simulink model "CSTD1_ClosedLoopLQG"  (Simulink 8.9)
settings: Solver=ode5  StartTime=0.0  StopTime=15  FixedStep=0.001  RelTol=1e-3  EnableMultiTasking=on
values from neighbouring files (symbols this model uses):
  dist_on = 1    [CSTD1_LQGdesign.m]
  F = zeros(1,6)    [CSTD1_LQGdesign.m]
  F2 = Fi(1:6)    [CSTD1_LQGdesign.m]
  Ki = Fi(7)    [CSTD1_LQGdesign.m]
  L = -lqr(A',C3',Q_lqe,R_lqe)'    [CSTD1_LQGdesign.m]
  LQG_activation = 0    [CSTD1_LQGdesign.m]
  pre_v = 0    [CSTD1_LQGdesign.m]
undefined symbols (not defined in the file or in its folder): A, B, C, D
libraries: simulink x1
settings Model: Creator=jb  LastModifiedBy=AMG
settings DataIOCC: ExternalInput=[t, Plant_input_u]  LimitDataPoints=off  MaxDataPoints=20000  SaveOutput=off
settings OptimizationCC: BlockReduction=off  ExpressionDepthLimit=2147483647
settings DebuggingCC: SolverPrmCheckMsg=warning
settings ConfigComp: CovSFcnEnable=off

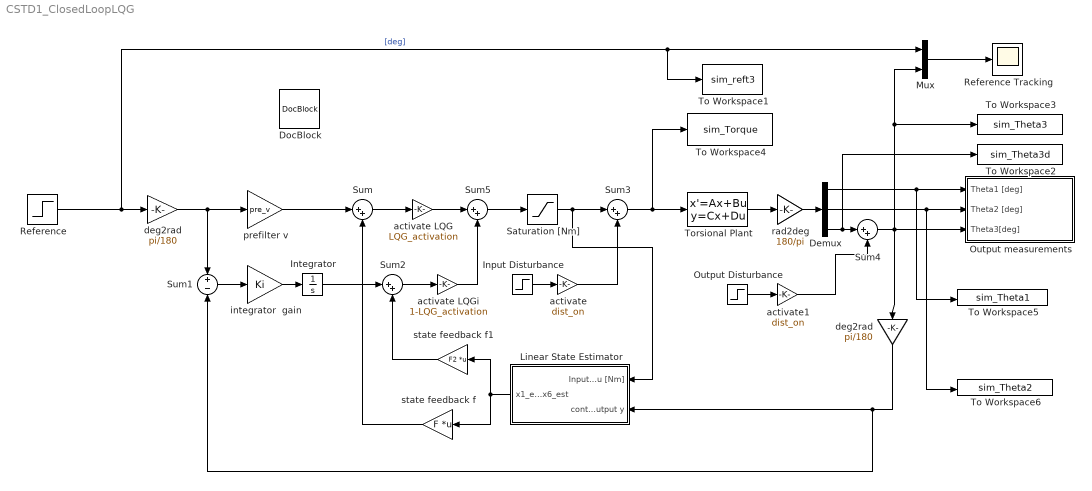
== system CSTD1_ClosedLoopLQG ==
  " deg2rad " : Gain  Gain=pi/180
  Demux : Demux  Outputs=3
  DocBlock : simulink/Model-Wide Utilities/DocBlock  DocumentType=Text
      content=|
      | % #########################################################################
      | % TUHH :: Institute for Control Systems :: Control Lab
      | % #########################################################################
      | % Experiment CSTD1: Control and Identification of a Torsional Plant
      | %
      | % Copyright Herbert Werner and Hamburg University of Technology, 2014
      | % #########################################################################
      | % This is the model containing the closed loop simulation for the LQG
      | % controllers design.
      | %
      | % Further, the following variables need to be in the workspace to run the
      | % experiment:
      | %  - pre_v   [double] : static prefilter
      | %  - F       [double] : standard state feedback gain
      | %  - L       [double] : observer gain
      | %  - F2      [double] : state feedback gain with integrator
      | %  - Ki      [double] : integrator gain
      | %  - A,B,C,D [double] : system matrices
      | %  - dist_on [double] : disturbance activation
      | %  - LQG_activation [double] : LQG switch
      | %
      | %----------------------------
      | % v.1.0 - 15-11-2014
      | % by Antonio Mendez G
  Input Disturbance : Step  Time=7  After=0.2  SampleTime=0
  Integrator : Integrator
  Linear State Estimator : Subsystem
  Mux : Mux  Inputs=2
  Output Disturbance : Step  Time=4  After=30  SampleTime=0
  Output measurements : Subsystem
  Reference : Step  Time=0  After=360  SampleTime=0
  Reference Tracking : Scope
  Saturation [Nm] : Saturate  UpperLimit=5*0.387  LowerLimit=-5*0.387
  Sum{,2..5} (5 alike) : Sum  Inputs=|++
  Sum1 : Sum  Inputs=+-
  To Workspace1 : ToWorkspace  VariableName=sim_reft3  SampleTime=-1
  To Workspace2 : ToWorkspace  VariableName=sim_Theta3d  SampleTime=-1
  To Workspace3 : ToWorkspace  VariableName=sim_Theta3  SampleTime=-1
  To Workspace4 : ToWorkspace  VariableName=sim_Torque  SampleTime=-1
  To Workspace5 : ToWorkspace  VariableName=sim_Theta1  SampleTime=-1
  To Workspace6 : ToWorkspace  VariableName=sim_Theta2  SampleTime=-1
  Torsional Plant : StateSpace  A=A  B=B  C=C  D=D  X0=[0 0.1 0 0.2 0 0.2]
  activate : Gain  Gain=dist_on
  activate LQG : Gain  Gain=LQG_activation
  activate LQGi : Gain  Gain=1-LQG_activation
  activate1 : Gain  Gain=dist_on
  deg2rad : Gain  Gain=pi/180
  integrator  gain : Gain  Gain=Ki
  prefilter v : Gain  Gain=pre_v
  rad2deg : Gain  Gain=180/pi
  state feedback f : Gain  Gain=F  Multiplication=Matrix(K*u) (u vector)
  state feedback f1 : Gain  Gain=F2  Multiplication=Matrix(K*u) (u vector)
  wires:
  Linear State Estimator/1(x1_est...x6_est) -> state feedback f1/1, state feedback f/1
  " deg2rad "/1 -> prefilter v/1, Sum1/1
  Reference/1 -> " deg2rad "/1, To Workspace1/1, Mux/1  "[deg]"
  rad2deg/1 -> Demux/1
  Torsional Plant/1 -> rad2deg/1
  state feedback f/1 -> Sum/2
  Mux/1 -> Reference Tracking/1
  Demux/2 -> To Workspace6/1, Output measurements/2(Theta2 [deg])
  Sum1/1 -> integrator  gain/1
  integrator  gain/1 -> Integrator/1
  deg2rad/1 -> Sum1/2, Linear State Estimator/2(control output y)
  Sum/1 -> activate LQG/1
  Integrator/1 -> Sum2/1
  state feedback f1/1 -> Sum2/2
  Sum2/1 -> activate LQGi/1
  Demux/1 -> To Workspace5/1, Output measurements/1(Theta1 [deg])
  Sum3/1 -> Torsional Plant/1, To Workspace4/1
  Saturation [Nm]/1 -> Linear State Estimator/1(Input u [Nm]), Sum3/1
  Output Disturbance/1 -> activate1/1
  Input Disturbance/1 -> activate/1
  activate/1 -> Sum3/2
  activate LQG/1 -> Sum5/1
  activate LQGi/1 -> Sum5/2
  Sum5/1 -> Saturation [Nm]/1
  prefilter v/1 -> Sum/1
  activate1/1 -> Sum4/2
  Demux/3 -> To Workspace2/1, Sum4/1
  Sum4/1 -> deg2rad/1, To Workspace3/1, Mux/2, Output measurements/3(Theta3[deg])

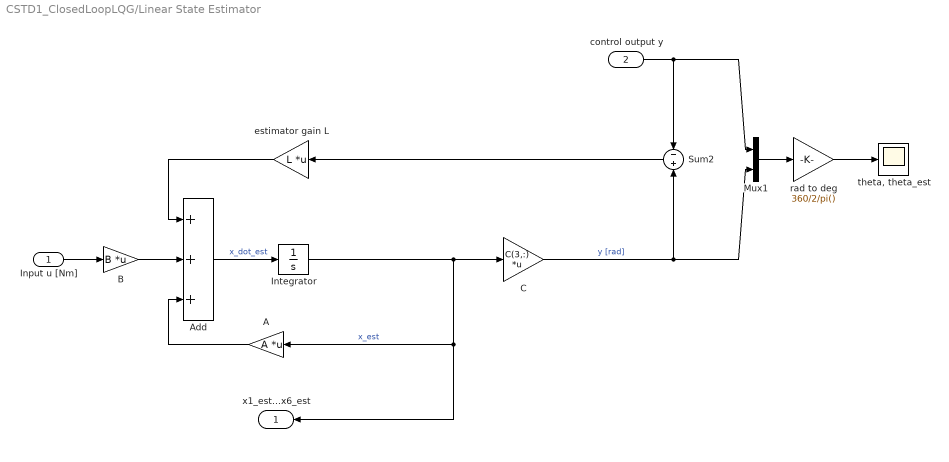
== system CSTD1_ClosedLoopLQG/Linear State Estimator ==
  Input u [Nm] : Inport
  control output y : Inport  Port=2
  " estimator gain L" : Gain  Gain=L  Multiplication=Matrix(K*u) (u vector)
  A : Gain  Gain=A  Multiplication=Matrix(K*u) (u vector)
  Add : Sum  Inputs=+++
  B : Gain  Gain=B  Multiplication=Matrix(K*u) (u vector)
  C : Gain  Gain=C(3,:)  Multiplication=Matrix(K*u) (u vector)
  Integrator : Integrator
  Mux1 : Mux  Inputs=2
  Sum2 : Sum  Inputs=-|+
  rad to deg : Gain  Gain=360/2/pi()
  "theta, theta_est" : Scope
  x1_est...x6_est : Outport
  wires:
  Input u [Nm]/1 -> B/1
  control output y/1 -> Sum2/1, Mux1/1
  Add/1 -> Integrator/1  "x_dot_est"
  Integrator/1 -> C/1, x1_est...x6_est/1, A/1  "x_est"
  C/1 -> Sum2/2, Mux1/2  "y [rad]"
  Mux1/1 -> rad to deg/1
  rad to deg/1 -> "theta, theta_est"/1
  " estimator gain L"/1 -> Add/1
  B/1 -> Add/2
  A/1 -> Add/3
  Sum2/1 -> " estimator gain L"/1

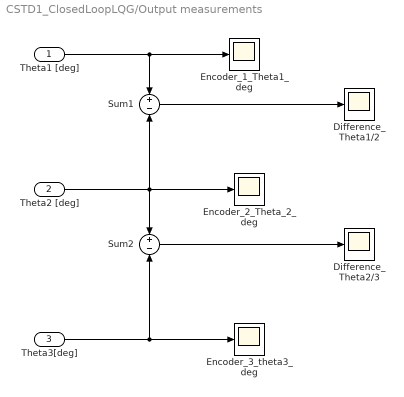
== system CSTD1_ClosedLoopLQG/Output measurements ==
  Theta1 [deg] : Inport
  Theta2 [deg] : Inport  Port=2
  Theta3[deg] : Inport  Port=3
  Difference_Theta1/2 : Scope
  Difference_Theta2/3 : Scope
  Encoder_1_Theta1_deg : Scope
  Encoder_2_Theta_2_deg : Scope
  Encoder_3_theta3_deg : Scope
  Sum1 : Sum  Inputs=+-
  Sum2 : Sum  Inputs=+-
  wires:
  Theta1 [deg]/1 -> Encoder_1_Theta1_deg/1, Sum1/1
  Theta3[deg]/1 -> Encoder_3_theta3_deg/1, Sum2/2
  Sum1/1 -> Difference_Theta1/2/1
  Sum2/1 -> Difference_Theta2/3/1
  Theta2 [deg]/1 -> Sum1/2, Encoder_2_Theta_2_deg/1, Sum2/1
